simulink model "test_parallel"  (R2013a)
settings: Solver=ode45  StartTime=0.0  StopTime=inf  RelTol=1e-3
settings Model: Creator=michelr  LastModifiedBy=michelr

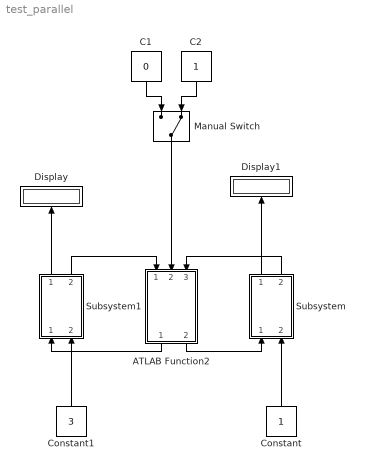
== system test_parallel ==
  ATLAB Function2 : MATLAB Function  TreatAsAtomicUnit=on
  C1 : Constant  Value=0
  C2 : Constant
  Constant : Constant
  Constant1 : Constant  Value=3
  Display : Display
  Display1 : Display
  Manual Switch : ManualSwitch  CurrentSetting=0
  Subsystem : Subsystem
  Subsystem1 : Subsystem
  wires:
  C1/1 -> Manual Switch/1
  C2/1 -> Manual Switch/2
  Manual Switch/1 -> ATLAB Function2/2(control)
  Constant1/1 -> Subsystem1/2(dataIn)
  Subsystem1/2(busOut) -> ATLAB Function2/1(busInA)
  ATLAB Function2/1(busOutA) -> Subsystem1/1(busIn)
  Constant/1 -> Subsystem/2(dataIn)
  Subsystem/1(dataOut) -> Display1/1
  Subsystem1/1(dataOut) -> Display/1
  Subsystem/2(busOut) -> ATLAB Function2/3(busInB)
  ATLAB Function2/2(busOutB) -> Subsystem/1(busIn)

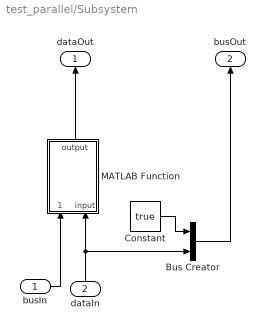
== system test_parallel/Subsystem ==
  busIn : Inport
  dataIn : Inport  Port=2
  Bus Creator : BusCreator  Inputs=2  OutDataTypeStr=Bus: breakerBus  NonVirtualBus=on
  Constant : Constant  Value=true
  MATLAB Function : MATLAB Function  TreatAsAtomicUnit=on
  dataOut : Outport
  busOut : Outport  Port=2  OutDataTypeStr=Bus: breakerBus
  wires:
  MATLAB Function/1(output) -> dataOut/1
  dataIn/1 -> Bus Creator/2, MATLAB Function/2(input)
  busIn/1 -> MATLAB Function/1(busIn)
  Bus Creator/1 -> busOut/1
  Constant/1 -> Bus Creator/1

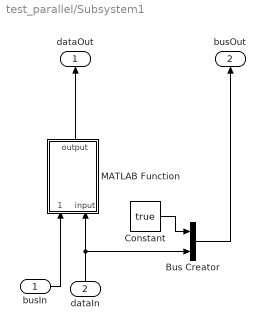
== system test_parallel/Subsystem1 ==
  busIn : Inport
  dataIn : Inport  Port=2
  Bus Creator : BusCreator  Inputs=2  OutDataTypeStr=Bus: breakerBus  NonVirtualBus=on
  Constant : Constant  Value=true
  MATLAB Function : MATLAB Function  TreatAsAtomicUnit=on
  dataOut : Outport
  busOut : Outport  Port=2  OutDataTypeStr=Bus: breakerBus
  wires:
  Constant/1 -> Bus Creator/1
  Bus Creator/1 -> busOut/1
  busIn/1 -> MATLAB Function/1(busIn)
  dataIn/1 -> MATLAB Function/2(input), Bus Creator/2
  MATLAB Function/1(output) -> dataOut/1

== matlab function test_parallel/Subsystem1/MATLAB Function ==
  data: output output; busIn input Bus: breakerBus; input input
function output = fcn(busIn,input)

if busIn.breaker == true
    output = mean([input busIn.data]);
else
    output = input;
end

== matlab function test_parallel/Subsystem/MATLAB Function ==
  data: output output; busIn input Bus: breakerBus; input input
function output = fcn(busIn,input)

if busIn.breaker == true
    output = mean([input busIn.data]);
else
    output = input;
end

== matlab function test_parallel/ATLAB Function2 ==
  data: busOutA output Bus: breakerBus; busOutB output Bus: breakerBus; busInA input Bus: breakerBus; control input; busInB input Bus: breakerBus
function [busOutA,busOutB] = fcn(busInA,control,busInB)

busOutA = busInB;
busOutB = busInA;

if (control*busInA.breaker*busInB.breaker == true)
    busOutA.breaker = true;
    busOutB.breaker = true;
else
    busOutA.breaker = false;
    busOutB.breaker = false;
end

end
